simulink model "control_system_final"  (R2024b)
settings: Solver=ode1  StartTime=0.0  StopTime=10.0  FixedStep=0.01  RelTol=1e-3
undefined symbols (not defined in the file): Total_Dist
settings Model: ExtModeTrigDuration=100  Creator=purple  LastModifiedBy=purple

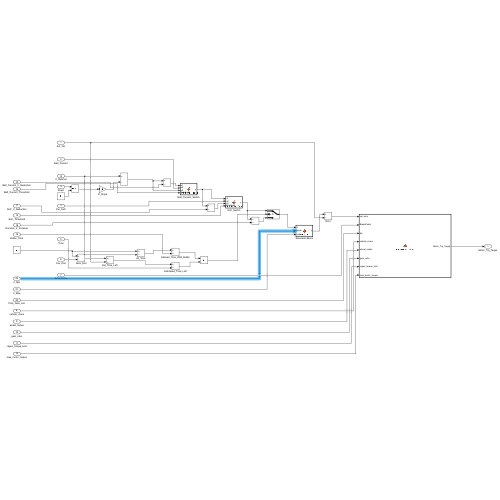
[thumbnail: Simulink's stored preview of the top-level diagram]
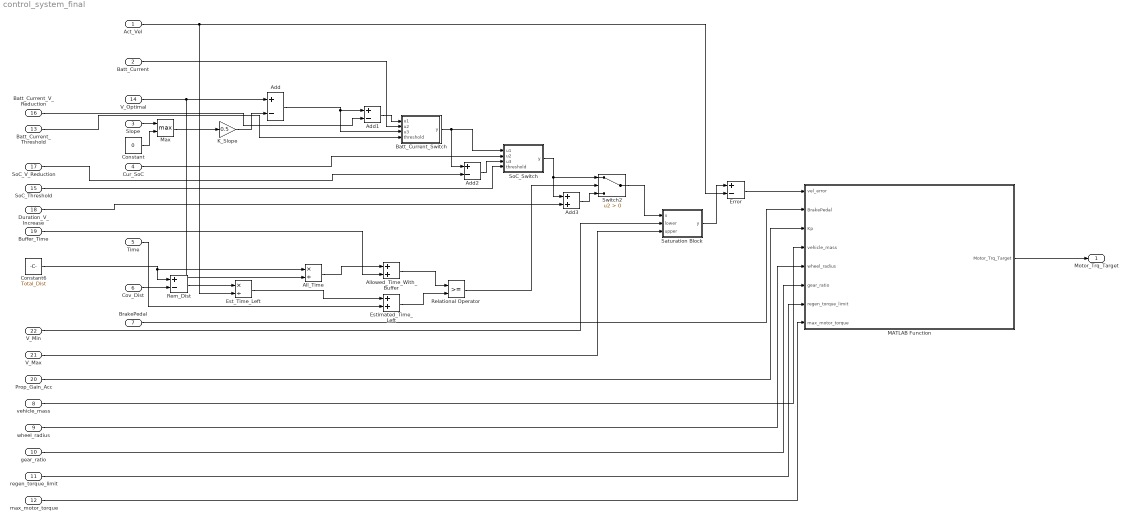
== system control_system_final ==
  Act_Vel : Inport
  Batt_Current : Inport  Port=2
  Slope : Inport  Port=3
  Cur_SoC : Inport  Port=4
  Time : Inport  Port=5
  Cov_Dist : Inport  Port=6
  BrakePedal : Inport  Port=7
  vehicle_mass : Inport  Port=8
  wheel_radius : Inport  Port=9
  gear_ratio : Inport  Port=10
  regen_torque_limit : Inport  Port=11
  max_motor_torque : Inport  Port=12
  Batt_Current_Threshold : Inport  Port=13
  V_Optimal : Inport  Port=14
  SoC_Threshold : Inport  Port=15
  Batt_Current_V_Reduction : Inport  Port=16
  SoC_V_Reduction : Inport  Port=17
  Duration_V_Increase : Inport  Port=18
  Buffer_Time : Inport  Port=19
  Prop_Gain_Acc : Inport  Port=20
  V_Max : Inport  Port=21
  V_Min : Inport  Port=22
  Add : Sum  Inputs=+-
  Add1 : Sum  Inputs=+-
  Add2 : Sum  Inputs=+-
  Add3 : Sum
  All_Time : Product  Inputs=*/
  Allowed_Time_With_Buffer : Sum
  Batt_Current_Switch : MATLAB Function  TreatAsAtomicUnit=on
  Constant : Constant  Value=0
  Constant6 : Constant  Value=Total_Dist
  Error : Sum  Inputs=+-
  Est_Time_Left : Product  Inputs=*/
  Estimated_Time_Left : Sum
  K_Slope : Gain  Gain=0.5
  MATLAB Function : MATLAB Function  TreatAsAtomicUnit=on
  Max : MinMax  Function=max  Inputs=2
  Relational Operator : RelationalOperator  OutDataTypeStr=boolean  RndMeth=Simplest  InputSameDT=off
  Rem_Dist : Sum  Inputs=+-
  Saturation Block : MATLAB Function  TreatAsAtomicUnit=on
  SoC_Switch : MATLAB Function  TreatAsAtomicUnit=on
  Switch2 : Switch  Criteria=u2 > Threshold  SaturateOnIntegerOverflow=off  InputSameDT=off
  Motor_Trq_Target : Outport
  wires:
  V_Optimal/1 -> All_Time/2, Add/1
  Slope/1 -> Max/1
  K_Slope/1 -> Add/2
  Constant/1 -> Max/2
  Max/1 -> K_Slope/1
  Add/1 -> Batt_Current_Switch/3(u3), Add1/1
  Batt_Current_V_Reduction/1 -> Add1/2
  Add1/1 -> Batt_Current_Switch/1(u1)
  Batt_Current/1 -> Batt_Current_Switch/2(u2)
  Cur_SoC/1 -> SoC_Switch/2(u2)
  Add2/1 -> SoC_Switch/3(u3)
  SoC_V_Reduction/1 -> Add2/2
  Constant6/1 -> Rem_Dist/1, All_Time/1
  Cov_Dist/1 -> Rem_Dist/2
  Rem_Dist/1 -> Est_Time_Left/1
  Act_Vel/1 -> Est_Time_Left/2, Error/2
  Est_Time_Left/1 -> Estimated_Time_Left/1
  All_Time/1 -> Allowed_Time_With_Buffer/1
  Buffer_Time/1 -> Allowed_Time_With_Buffer/2
  Time/1 -> Estimated_Time_Left/2
  Allowed_Time_With_Buffer/1 -> Relational Operator/1
  Estimated_Time_Left/1 -> Relational Operator/2
  Relational Operator/1 -> Switch2/2
  Duration_V_Increase/1 -> Add3/2
  Add3/1 -> Switch2/3
  Switch2/1 -> Saturation Block/1(u)
  Saturation Block/1(y) -> Error/1
  Error/1 -> MATLAB Function/1(vel_error)
  BrakePedal/1 -> MATLAB Function/2(BrakePedal)
  MATLAB Function/1(Motor_Trq_Target) -> Motor_Trq_Target/1
  Prop_Gain_Acc/1 -> MATLAB Function/3(Kp)
  vehicle_mass/1 -> MATLAB Function/4(vehicle_mass)
  wheel_radius/1 -> MATLAB Function/5(wheel_radius)
  gear_ratio/1 -> MATLAB Function/6(gear_ratio)
  regen_torque_limit/1 -> MATLAB Function/7(regen_torque_limit)
  max_motor_torque/1 -> MATLAB Function/8(max_motor_torque)
  Batt_Current_Threshold/1 -> Batt_Current_Switch/4(threshold)
  Batt_Current_Switch/1(y) -> SoC_Switch/1(u1), Add2/1
  SoC_Threshold/1 -> SoC_Switch/4(threshold)
  SoC_Switch/1(y) -> Switch2/1, Add3/1
  V_Max/1 -> Saturation Block/3(upper)
  V_Min/1 -> Saturation Block/2(lower)

== matlab function control_system_final/Batt_Current_Switch ==
  data: u1 input; y output; u2 input; u3 input; threshold input
function y = conditional_pass(u1, u2, u3, threshold)
% Pass u1 when u2 >= threshold; otherwise, pass u3

% Inputs:
% u1 - Data input 1
% u2 - Control input
% u3 - Data input 3
% threshold - Comparison threshold

    if u2 >= threshold
        y = u1;
    else
        y = u3;
    end
end

== matlab function control_system_final/MATLAB Function ==
  data: vel_error input; Motor_Trq_Target output; BrakePedal input; Kp input; vehicle_mass input; wheel_radius input; gear_ratio input; regen_torque_limit input; max_motor_torque input
function Motor_Trq_Target = TorqueCalculator(...
    vel_error, BrakePedal, Kp, vehicle_mass, wheel_radius, ...
    gear_ratio, regen_torque_limit, max_motor_torque)

% Calculate motor torque target based on velocity error and vehicle parameters
%
% Inputs:
%   vel_error           - Velocity error (Trgt_Vel - Act_Vel) [m/s]
%   BrakePedal          - Brake pedal status (0–1 or 0–100) [scalar]
%   Kp                  - Proportional gain for accel (m/s² per m/s error)
%   vehicle_mass        - Vehicle mass (kg)
%   wheel_radius        - Wheel radius (m)
%   gear_ratio          - Gear ratio (dimensionless)
%   regen_torque_limit  - Max regenerative braking torque (negative Nm)
%   max_motor_torque    - Maximum motor torque (positive Nm)
%
% Output:
%   Motor_Trq_Target    - Target motor torque (Nm)

% Step 1: Desired acceleration from velocity error
desired_accel = Kp * vel_error; % m/s²

% Step 2: Required force
required_force = vehicle_mass * desired_accel; % Newtons

% Step 3: Torque at wheel
torque_at_wheel = required_force * wheel_radius; % Nm

% Step 4: Back-calculate motor torque via gear ratio
motor_torque = torque_at_wheel / gear_ratio; % Nm

% Step 5: Conditional torque switching with blended regen
if (BrakePedal > 0) || (vel_error < 0)
    % Normalize BrakePedal if needed (e.g., convert 0–100 to 0–1)
    if BrakePedal > 1
        BrakePedal = BrakePedal / 100;
    end
    
    % Calculate scaled regenerative torque
    regen_torque = BrakePedal * regen_torque_limit;  % Will be negative

    % Select the higher of regen torque or computed torque (more conservative)
    Motor_Trq_Target = max(motor_torque, regen_torque);
else
    % No braking needed — use calculated positive torque
    Motor_Trq_Target = motor_torque;
end

% Step 6: Clamp final torque within motor safety limits
Motor_Trq_Target = min(max(Motor_Trq_Target, regen_torque_limit), max_motor_torque);

end

== matlab function control_system_final/SoC_Switch ==
  data: u1 input; y output; u2 input; u3 input; threshold input
function y = conditional_pass(u1, u2, u3, threshold)
% Pass u1 when u2 >= threshold; otherwise, pass u3

% Inputs:
% u1 - Data input 1
% u2 - Control input
% u3 - Data input 3
% threshold - Comparison threshold

    if u2 >= threshold
        y = u1;
    else
        y = u3;
    end
end

== matlab function control_system_final/Saturation Block ==
  data: u input; y output; lower input; upper input
function y = saturate(u, lower, upper)
% Limit the input signal u between lower and upper bounds

% Inputs:
% u     - input signal
% lower - lower saturation limit
% upper - upper saturation limit

    if u < lower
        y = lower;
    elseif u > upper
        y = upper;
    else
        y = u;
    end
end
